simulink model "board_audio"  (R2024b)
settings: Solver=FixedStepDiscrete  StartTime=0.0  StopTime=10.0  FixedStep=Ts  RelTol=1e-3
PreLoadFcn:
  | if ~exist('b','var'), iir_setup; end
values from neighbouring files (symbols this model uses):
  Ts = 1/Fs    (= 2.08333333333e-05)    [iir_setup.m]
libraries: dspsrcs4 x1
settings Model: Creator=samue  LastModifiedBy=samue
settings DebuggingCC: IntegerOverflowMsg=none  ParameterPrecisionLossMsg=none

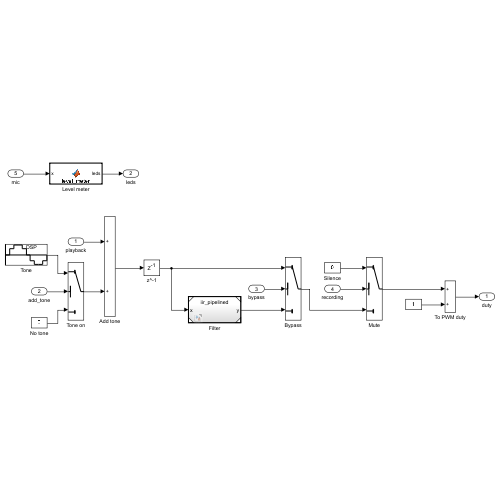
[thumbnail: Simulink's stored preview of the top-level diagram]
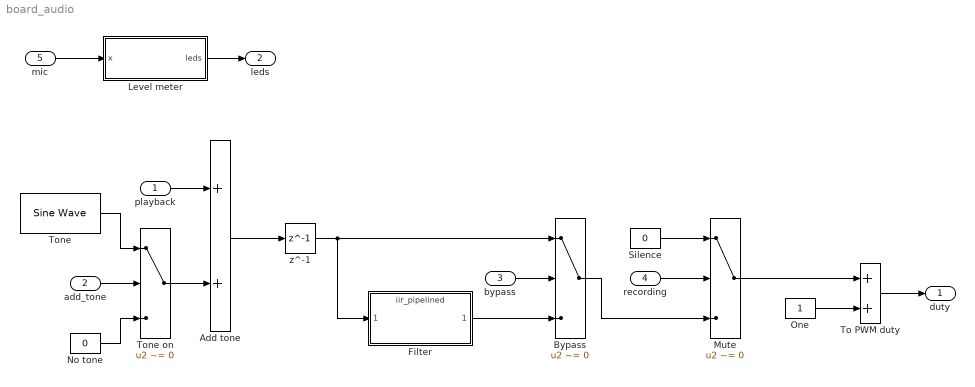
== system board_audio ==
  playback : Inport  OutDataTypeStr=InT  SampleTime=Ts
  add_tone : Inport  Port=2  OutDataTypeStr=boolean  SampleTime=Ts
  bypass : Inport  Port=3  OutDataTypeStr=boolean  SampleTime=Ts
  recording : Inport  Port=4  OutDataTypeStr=boolean  SampleTime=Ts
  mic : Inport  Port=5  OutDataTypeStr=InT  SampleTime=Ts
  Add tone : Sum  OutDataTypeStr=InT  SaturateOnIntegerOverflow=on
  Bypass : Switch  Criteria=u2 ~= 0  SaturateOnIntegerOverflow=off  InputSameDT=off
  Filter : ModelReference  ModelNameDialog=iir_pipelined  SimulationMode=Normal  ModelReferenceVersion=1.3
  Level meter : MATLAB Function  TreatAsAtomicUnit=on
  Mute : Switch  Criteria=u2 ~= 0  SaturateOnIntegerOverflow=off  InputSameDT=off
  No tone : Constant  Value=0  OutDataTypeStr=InT
  One : Constant  OutDataTypeStr=fixdt(0,1,0)
  Silence : Constant  Value=0  OutDataTypeStr=InT
  To PWM duty : Sum  OutDataTypeStr=fixdt(0,11,10)
  Tone : dspsrcs4/Sine Wave  Amplitude=1/8  Frequency=4800  Phase=0  SampleMode=Discrete  OutComplex=Real  CompMethod=Table lookup  TableSize=Speed  SampleTime=Ts  SamplesPerFrame=1  ResetState=Restart at time zero  OutputFrames=off  dataType=User-defined  wordLen=16  udDataType=InT  fracBitsMode=Best precision  numFracBits=0  OutDataTypeStr=fixdt(1,16,15)  LastOutDataTypeStr=fixdt(1,16,15)
  Tone on : Switch  Criteria=u2 ~= 0  SaturateOnIntegerOverflow=off  InputSameDT=off
  z^-1 : Delay  DelayLength=1
  duty : Outport
  leds : Outport  Port=2
  wires:
  mic/1 -> Level meter/1(x)
  add_tone/1 -> Tone on/2
  Level meter/1(leds) -> leds/1
  z^-1/1 -> Filter/1, Bypass/1
  No tone/1 -> Tone on/3
  Filter/1 -> Bypass/3
  playback/1 -> Add tone/1
  Add tone/1 -> z^-1/1
  Tone on/1 -> Add tone/2
  bypass/1 -> Bypass/2
  Silence/1 -> Mute/1
  recording/1 -> Mute/2
  Bypass/1 -> Mute/3
  Mute/1 -> To PWM duty/1
  One/1 -> To PWM duty/2
  To PWM duty/1 -> duty/1
  Tone/1 -> Tone on/1

== matlab function board_audio/Level meter ==
  data: x input; leds output
function leds = level_meter(x)
% Peak level of x over each 8192 samples (0.17 s) represented on LED bar
persistent peak held count
if isempty(peak)
    peak  = fi(0, 0, 16, 15);
    held  = fi(0, 0, 16, 15);
    count = fi(0, 0, 13, 0, 'OverflowAction', 'Wrap');
end
a = fi(abs(x), 0, 16, 15);
if count == 0
    held(:) = peak;
    peak(:) = a;
elseif a > peak
    peak(:) = a;
end
count(:) = count + 1;

leds = fi(0, 0, 15, 0);
for k = coder.unroll(1:15)                % one comparator per LED
    if held >= 2^(k-16)
        leds = bitset(leds, k, 1);
    end
end
